simulink library "NAV420Lib"  (Simulink 7.4)
settings: Solver=ode45  StartTime=0.0  StopTime=10.0  RelTol=1e-3
libraries: simulink x25, NAV420Lib x9
settings Model: Creator=djulzz  LastModifiedBy=djulzz

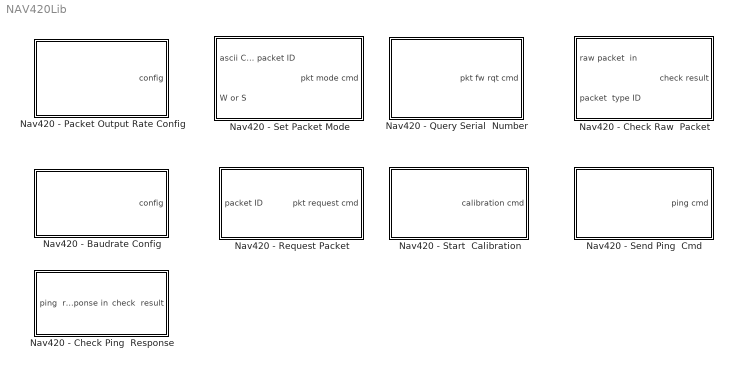
== system NAV420Lib ==
  Nav420 - Baudrate Config : Subsystem  mask{baudrateIndex=9600, SaveConfig=off}
      mask prompts: baudrateIndex "Select the Baudrate (Bauds)"; SaveConfig "Check if the config is to be used at next startup"
      mask StyleString: popup(9600|19200|38400|57600),checkbox
  Nav420 - Check Ping  Response : Subsystem
  Nav420 - Check Raw  Packet : Subsystem
  Nav420 - Packet Output Rate Config : Subsystem  mask{shouldSave=off, output_rate=100}
      mask prompts: shouldSave "Save Ouput Rate for Next Bootup?"; output_rate "Output Rate (Hz)"
      mask StyleString: checkbox,popup(0|2|10|20|25|50|100)
  Nav420 - Query Serial  Number : Subsystem
  Nav420 - Request Packet : Subsystem
  Nav420 - Send Ping  Cmd : Subsystem
  Nav420 - Set Packet Mode : Subsystem
  Nav420 - Start  Calibration : Subsystem

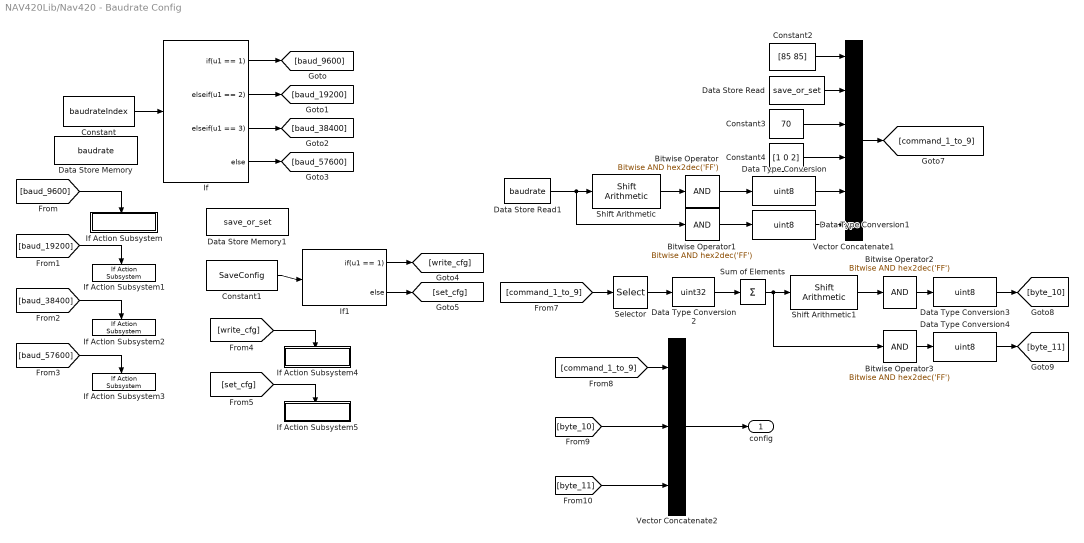
== system NAV420Lib/Nav420 - Baudrate Config ==
  Bitwise Operator{,1..3} (4 alike) : simulink/Logic and Bit Operations/Bitwise Operator  logicop=AND  UseBitMask=on  BitMask=hex2dec('FF')  BitMaskRealWorld=Stored Integer
  Constant : Constant  Value=baudrateIndex  OutDataTypeMode=uint8  OutDataType=fixdt(1, 16)  OutScaling=2^0  OutDataTypeStr=uint8  SampleTime=-1
  Constant1 : Constant  Value=SaveConfig  OutDataTypeMode=uint8  OutDataType=fixdt(1, 16)  OutScaling=2^0  OutDataTypeStr=uint8  SampleTime=-1
  Constant2 : Constant  Value=[85 85]  OutDataTypeMode=uint8  OutDataType=fixdt(1, 16)  OutScaling=2^0  OutDataTypeStr=uint8  SampleTime=-1
  Constant3 : Constant  Value=70  OutDataTypeMode=uint8  OutDataType=fixdt(1, 16)  OutScaling=2^0  OutDataTypeStr=uint8  SampleTime=-1
  Constant4 : Constant  Value=[1 0 2]  OutDataTypeMode=uint8  OutDataType=fixdt(1, 16)  OutScaling=2^0  OutDataTypeStr=uint8  SampleTime=-1
  Data Store Memory : DataStoreMemory  DataStoreName=baudrate  DataType=uint32  OutDataType=fixdt(1, 16)  OutScaling=2^0  OutDataTypeStr=uint32
  Data Store Memory1 : DataStoreMemory  DataStoreName=save_or_set  DataType=uint8  OutDataType=fixdt(1, 16)  OutScaling=2^0  OutDataTypeStr=uint8
  Data Store Read : DataStoreRead  DataStoreName=save_or_set  SampleTime=-1
  Data Store Read1 : DataStoreRead  DataStoreName=baudrate  SampleTime=0
  Data Type Conversion{,1,3..4} (4 alike) : DataTypeConversion  OutDataTypeMode=uint8  OutDataType=fixdt(1, 16)  OutScaling=2^0  OutDataTypeStr=uint8  RndMeth=Nearest
  Data Type Conversion2 : DataTypeConversion  OutDataTypeMode=uint32  OutDataType=fixdt(1, 16)  OutScaling=2^0  OutDataTypeStr=uint32  RndMeth=Nearest
  If : If  IfExpression=u1 == 1  ElseIfExpressions=u1 == 2, u1 == 3
  If Action Subsystem : Subsystem  TreatAsAtomicUnit=on
  If Action Subsystem1 : NAV420Lib/Nav420 - Baudrate Config/If Action Subsystem  SystemSampleTime=-1
      link override Constant: Value=1
      link override Data Store Write: DataStoreName=baudrate
  If Action Subsystem2 : NAV420Lib/Nav420 - Baudrate Config/If Action Subsystem  SystemSampleTime=-1
      link override Constant: Value=2
      link override Data Store Write: DataStoreName=baudrate
  If Action Subsystem3 : NAV420Lib/Nav420 - Baudrate Config/If Action Subsystem  SystemSampleTime=-1
      link override Constant: Value=3
      link override Data Store Write: DataStoreName=baudrate
  If Action Subsystem4 : Subsystem  AncestorBlock=|  TreatAsAtomicUnit=on
      | NAV420Lib/Nav420 - Baudrate
      | Config/If Action
      | Subsystem
  If Action Subsystem5 : Subsystem  AncestorBlock=|  TreatAsAtomicUnit=on
      | NAV420Lib/Nav420 - Baudrate
      | Config/If Action
      | Subsystem
  If1 : If  IfExpression=u1 == 1
  Selector : Selector  InputPortWidth=9  IndexOptions=Index vector (dialog)  Indices=[3 4 5 6 7 8 9]  OutputSizes=1
  Shift Arithmetic : simulink/Logic and Bit Operations/Shift Arithmetic  SystemSampleTime=-1  nBitShiftRight=8  nBinPtShiftRight=0
  Shift Arithmetic1 : simulink/Logic and Bit Operations/Shift Arithmetic  SystemSampleTime=-1  nBitShiftRight=8  nBinPtShiftRight=0
  Sum of Elements : Sum  Inputs=+  OutDataType=fixdt(1, 16)  OutScaling=2^-10
  Vector Concatenate1 : Concatenate  NumInputs=6  Mode=Vector
  Vector Concatenate2 : Concatenate  NumInputs=3  Mode=Vector
  config : Outport  DataType=uint8  OutDataType=fixdt(1, 16)  OutScaling=2^0  OutDataTypeStr=uint8
  wires:
  Constant/1 -> If/1
  If/1 -> [baud_9600]
  If/2 -> [baud_19200]
  If/3 -> [baud_38400]
  If/4 -> [baud_57600]
  [baud_9600] -> If Action Subsystem/Action
  [baud_19200] -> If Action Subsystem1/Action
  [baud_38400] -> If Action Subsystem2/Action
  [baud_57600] -> If Action Subsystem3/Action
  Data Store Read1/1 -> Shift Arithmetic/1, Bitwise Operator1/1
  Shift Arithmetic/1 -> Bitwise Operator/1
  Bitwise Operator1/1 -> Data Type Conversion1/1
  Bitwise Operator/1 -> Data Type Conversion/1
  Constant1/1 -> If1/1
  If1/2 -> [set_cfg]
  If1/1 -> [write_cfg]
  [write_cfg] -> If Action Subsystem4/Action
  [set_cfg] -> If Action Subsystem5/Action
  Constant2/1 -> Vector Concatenate1/1
  Data Store Read/1 -> Vector Concatenate1/2
  Constant3/1 -> Vector Concatenate1/3
  Constant4/1 -> Vector Concatenate1/4
  Data Type Conversion/1 -> Vector Concatenate1/5
  Data Type Conversion1/1 -> Vector Concatenate1/6
  Vector Concatenate1/1 -> [command_1_to_9]
  Selector/1 -> Data Type Conversion2/1
  Data Type Conversion2/1 -> Sum of Elements/1
  Shift Arithmetic1/1 -> Bitwise Operator2/1
  Bitwise Operator2/1 -> Data Type Conversion3/1
  Sum of Elements/1 -> Shift Arithmetic1/1, Bitwise Operator3/1
  [command_1_to_9] -> Selector/1
  Data Type Conversion3/1 -> [byte_10]
  Bitwise Operator3/1 -> Data Type Conversion4/1
  Data Type Conversion4/1 -> [byte_11]
  [command_1_to_9] -> Vector Concatenate2/1
  [byte_10] -> Vector Concatenate2/2
  [byte_11] -> Vector Concatenate2/3
  Vector Concatenate2/1 -> config/1

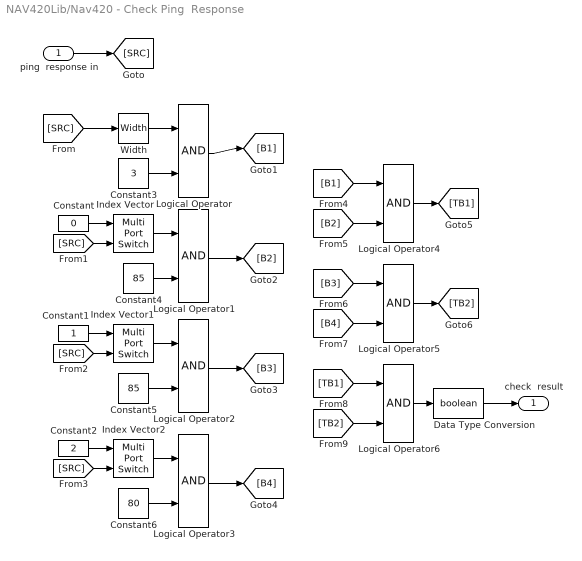
== system NAV420Lib/Nav420 - Check Ping  Response ==
  ping  response in : Inport  DataType=uint8  OutDataType=fixdt(1, 16)  OutScaling=2^0  OutDataTypeStr=uint8
  Constant : Constant  Value=0  OutDataType=fixdt(1, 16)  OutScaling=2^0  SampleTime=-1
  Constant1 : Constant  OutDataType=fixdt(1, 16)  OutScaling=2^0  SampleTime=-1
  Constant2 : Constant  Value=2  OutDataType=fixdt(1, 16)  OutScaling=2^0  SampleTime=-1
  Constant3 : Constant  Value=3  OutDataTypeMode=uint8  OutDataType=fixdt(1, 16)  OutScaling=2^0  OutDataTypeStr=uint8  SampleTime=-1
  Constant4 : Constant  Value=85  OutDataTypeMode=uint8  OutDataType=fixdt(1, 16)  OutScaling=2^0  OutDataTypeStr=uint8  SampleTime=-1
  Constant5 : Constant  Value=85  OutDataTypeMode=uint8  OutDataType=fixdt(1, 16)  OutScaling=2^0  OutDataTypeStr=uint8  SampleTime=-1
  Constant6 : Constant  Value=80  OutDataTypeMode=uint8  OutDataType=fixdt(1, 16)  OutScaling=2^0  OutDataTypeStr=uint8  SampleTime=-1
  Data Type Conversion : DataTypeConversion  OutDataTypeMode=boolean  OutDataType=fixdt(1, 16)  OutScaling=2^0  OutDataTypeStr=boolean
  Index Vector : MultiPortSwitch  Inputs=1  zeroidx=on  OutDataType=fixdt(1, 16)  OutScaling=2^0
  Index Vector1 : MultiPortSwitch  Inputs=1  zeroidx=on  OutDataType=fixdt(1, 16)  OutScaling=2^0
  Index Vector2 : MultiPortSwitch  Inputs=1  zeroidx=on  OutDataType=fixdt(1, 16)  OutScaling=2^0
  Logical Operator{,1..6} (7 alike) : Logic  AllPortsSameDT=off  OutDataTypeMode=boolean  LogicDataType=fixdt(0, 8)  OutDataTypeStr=boolean
  Width : Width
  check  result : Outport  DataType=boolean  OutDataType=fixdt(1, 16)  OutScaling=2^0  OutDataTypeStr=boolean
  wires:
  ping  response in/1 -> [SRC]
  [SRC] -> Width/1
  [SRC] -> Index Vector2/2
  [SRC] -> Index Vector1/2
  [SRC] -> Index Vector/2
  Constant/1 -> Index Vector/1
  Constant1/1 -> Index Vector1/1
  Constant2/1 -> Index Vector2/1
  Width/1 -> Logical Operator/1
  Constant3/1 -> Logical Operator/2
  Index Vector/1 -> Logical Operator1/1
  Constant4/1 -> Logical Operator1/2
  Constant5/1 -> Logical Operator2/2
  Index Vector1/1 -> Logical Operator2/1
  Constant6/1 -> Logical Operator3/2
  Index Vector2/1 -> Logical Operator3/1
  Logical Operator3/1 -> [B4]
  Logical Operator2/1 -> [B3]
  Logical Operator1/1 -> [B2]
  Logical Operator/1 -> [B1]
  [B2] -> Logical Operator4/2
  [B1] -> Logical Operator4/1
  [B4] -> Logical Operator5/2
  [B3] -> Logical Operator5/1
  Logical Operator5/1 -> [TB2]
  Logical Operator4/1 -> [TB1]
  [TB2] -> Logical Operator6/2
  [TB1] -> Logical Operator6/1
  Logical Operator6/1 -> Data Type Conversion/1
  Data Type Conversion/1 -> check  result/1

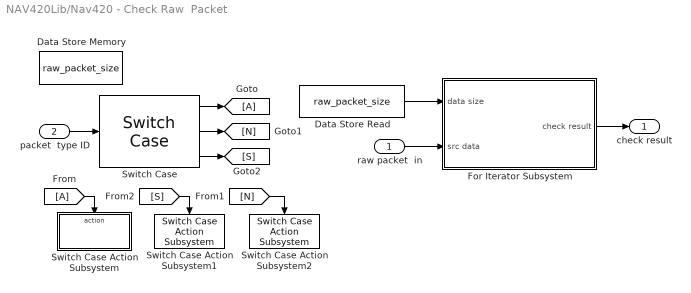
== system NAV420Lib/Nav420 - Check Raw  Packet ==
  raw packet  in : Inport  DataType=uint8  OutDataType=fixdt(1, 16)  OutScaling=2^0  OutDataTypeStr=uint8
  packet  type ID : Inport  Port=2  DataType=int8  OutDataType=fixdt(1, 16)  OutScaling=2^0  OutDataTypeStr=int8
  Data Store Memory : DataStoreMemory  DataStoreName=raw_packet_size  DataType=uint8  OutDataType=fixdt(1, 16)  OutScaling=2^0  OutDataTypeStr=uint8
  Data Store Read : DataStoreRead  DataStoreName=raw_packet_size  SampleTime=-1
  For Iterator Subsystem : Subsystem  TreatAsAtomicUnit=on
  Switch Case : SwitchCase  CaseConditions={65,78}
  Switch Case Action Subsystem : Subsystem  TreatAsAtomicUnit=on
  Switch Case Action Subsystem1 : NAV420Lib/Nav420 - Check Raw  Packet/Switch Case Action Subsystem  SystemSampleTime=-1
  Switch Case Action Subsystem2 : NAV420Lib/Nav420 - Check Raw  Packet/Switch Case Action Subsystem  SystemSampleTime=-1
      link override Constant: Value=37
  check result : Outport  DataType=boolean  OutDataType=fixdt(1, 16)  OutScaling=2^0  OutDataTypeStr=boolean
  wires:
  packet  type ID/1 -> Switch Case/1
  Switch Case/1 -> [A]
  Switch Case/2 -> [N]
  Switch Case/3 -> [S]
  [A] -> Switch Case Action Subsystem/Action
  [S] -> Switch Case Action Subsystem1/Action
  [N] -> Switch Case Action Subsystem2/Action
  Data Store Read/1 -> For Iterator Subsystem/1(data size)
  raw packet  in/1 -> For Iterator Subsystem/2(src data)
  For Iterator Subsystem/1(check result) -> check result/1

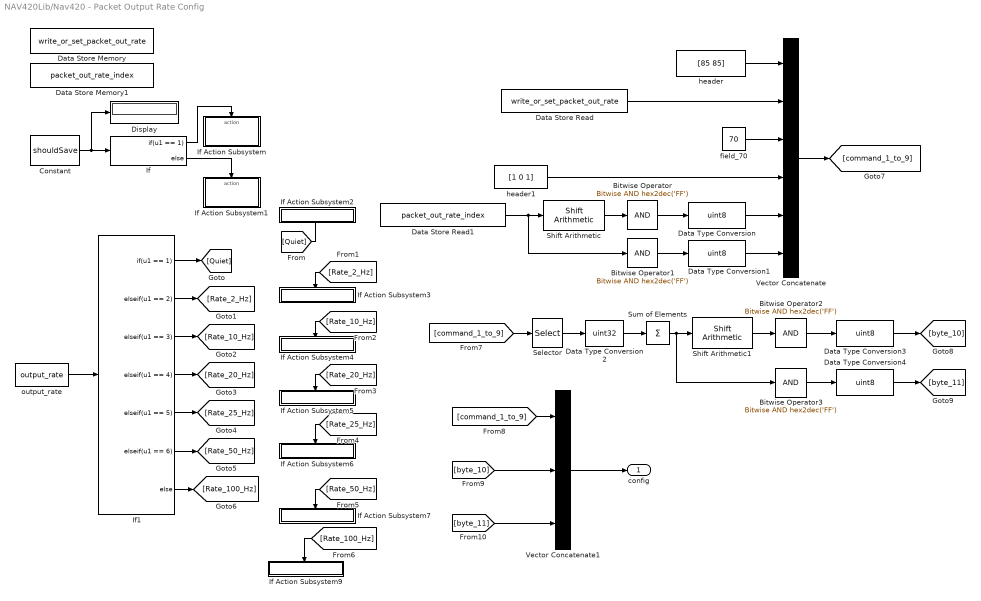
== system NAV420Lib/Nav420 - Packet Output Rate Config ==
  Bitwise Operator{,1..3} (4 alike) : simulink/Logic and Bit Operations/Bitwise Operator  logicop=AND  UseBitMask=on  BitMask=hex2dec('FF')  BitMaskRealWorld=Stored Integer
  Constant : Constant  Value=shouldSave  OutDataTypeMode=int32  OutDataType=fixdt(1, 16)  OutScaling=2^0  OutDataTypeStr=int32  SampleTime=-1
  Data Store Memory : DataStoreMemory  DataStoreName=write_or_set_packet_out_rate  DataType=uint8  OutDataType=fixdt(1, 16)  OutScaling=2^0  OutDataTypeStr=uint8
  Data Store Memory1 : DataStoreMemory  DataStoreName=packet_out_rate_index  DataType=uint8  OutDataType=fixdt(1, 16)  OutScaling=2^0  OutDataTypeStr=uint8
  Data Store Read : DataStoreRead  DataStoreName=write_or_set_packet_out_rate  SampleTime=-1
  Data Store Read1 : DataStoreRead  DataStoreName=packet_out_rate_index  SampleTime=-1
  Data Type Conversion{,1,3..4} (4 alike) : DataTypeConversion  OutDataTypeMode=uint8  OutDataType=fixdt(1, 16)  OutScaling=2^0  OutDataTypeStr=uint8  RndMeth=Nearest
  Data Type Conversion2 : DataTypeConversion  OutDataTypeMode=uint32  OutDataType=fixdt(1, 16)  OutScaling=2^0  OutDataTypeStr=uint32  RndMeth=Nearest
  Display : Display
  If : If  IfExpression=u1 == 1
  If Action Subsystem : Subsystem  TreatAsAtomicUnit=on
  If Action Subsystem1 : Subsystem  TreatAsAtomicUnit=on
  If Action Subsystem2 : Subsystem  TreatAsAtomicUnit=on
  If Action Subsystem3 : Subsystem  TreatAsAtomicUnit=on
  If Action Subsystem4 : Subsystem  TreatAsAtomicUnit=on
  If Action Subsystem5 : Subsystem  TreatAsAtomicUnit=on
  If Action Subsystem6 : Subsystem  TreatAsAtomicUnit=on
  If Action Subsystem7 : Subsystem  TreatAsAtomicUnit=on
  If Action Subsystem9 : Subsystem  TreatAsAtomicUnit=on
  If1 : If  IfExpression=u1 == 1  ElseIfExpressions=u1 == 2, u1 == 3, u1 == 4, u1 == 5, u1 == 6
  Selector : Selector  InputPortWidth=9  IndexOptions=Index vector (dialog)  Indices=[3 4 5 6 7 8 9]  OutputSizes=1
  Shift Arithmetic : simulink/Logic and Bit Operations/Shift Arithmetic  SystemSampleTime=-1  nBitShiftRight=8  nBinPtShiftRight=0
  Shift Arithmetic1 : simulink/Logic and Bit Operations/Shift Arithmetic  SystemSampleTime=-1  nBitShiftRight=8  nBinPtShiftRight=0
  Sum of Elements : Sum  Inputs=+  OutDataType=fixdt(1, 16)  OutScaling=2^-10
  Vector Concatenate : Concatenate  NumInputs=6  Mode=Vector
  Vector Concatenate1 : Concatenate  NumInputs=3  Mode=Vector
  field_70 : Constant  Value=70  OutDataTypeMode=uint8  OutDataType=fixdt(1, 16)  OutScaling=2^0  OutDataTypeStr=uint8  SampleTime=-1
  header : Constant  Value=[85 85]  OutDataTypeMode=uint8  OutDataType=fixdt(1, 16)  OutScaling=2^0  OutDataTypeStr=uint8  SampleTime=-1
  header1 : Constant  Value=[1 0 1]  OutDataTypeMode=uint8  OutDataType=fixdt(1, 16)  OutScaling=2^0  OutDataTypeStr=uint8  SampleTime=-1
  output_rate : Constant  Value=output_rate  OutDataTypeMode=uint8  OutDataType=fixdt(1, 16)  OutScaling=2^0  OutDataTypeStr=uint8  SampleTime=-1
  config : Outport  DataType=uint8  OutDataType=fixdt(1, 16)  OutScaling=2^0  OutDataTypeStr=uint8
  wires:
  Constant/1 -> If/1, Display/1
  If/2 -> If Action Subsystem1/Action
  header/1 -> Vector Concatenate/1
  If/1 -> If Action Subsystem/Action
  Data Store Read/1 -> Vector Concatenate/2
  field_70/1 -> Vector Concatenate/3
  header1/1 -> Vector Concatenate/4
  output_rate/1 -> If1/1
  Data Store Read1/1 -> Shift Arithmetic/1, Bitwise Operator1/1
  Shift Arithmetic/1 -> Bitwise Operator/1
  Bitwise Operator1/1 -> Data Type Conversion1/1
  Bitwise Operator/1 -> Data Type Conversion/1
  Data Type Conversion/1 -> Vector Concatenate/5
  Data Type Conversion1/1 -> Vector Concatenate/6
  If1/1 -> [Quiet]
  [Quiet] -> If Action Subsystem2/Action
  If1/2 -> [Rate_2_Hz]
  [Rate_2_Hz] -> If Action Subsystem3/Action
  If1/3 -> [Rate_10_Hz]
  [Rate_10_Hz] -> If Action Subsystem4/Action
  If1/4 -> [Rate_20_Hz]
  [Rate_20_Hz] -> If Action Subsystem5/Action
  If1/5 -> [Rate_25_Hz]
  [Rate_25_Hz] -> If Action Subsystem6/Action
  If1/6 -> [Rate_50_Hz]
  [Rate_50_Hz] -> If Action Subsystem7/Action
  If1/7 -> [Rate_100_Hz]
  [Rate_100_Hz] -> If Action Subsystem9/Action
  Selector/1 -> Data Type Conversion2/1
  Data Type Conversion2/1 -> Sum of Elements/1
  Shift Arithmetic1/1 -> Bitwise Operator2/1
  Bitwise Operator2/1 -> Data Type Conversion3/1
  Sum of Elements/1 -> Shift Arithmetic1/1, Bitwise Operator3/1
  Bitwise Operator3/1 -> Data Type Conversion4/1
  Vector Concatenate/1 -> [command_1_to_9]
  [command_1_to_9] -> Selector/1
  Data Type Conversion3/1 -> [byte_10]
  Data Type Conversion4/1 -> [byte_11]
  [command_1_to_9] -> Vector Concatenate1/1
  [byte_10] -> Vector Concatenate1/2
  [byte_11] -> Vector Concatenate1/3
  Vector Concatenate1/1 -> config/1

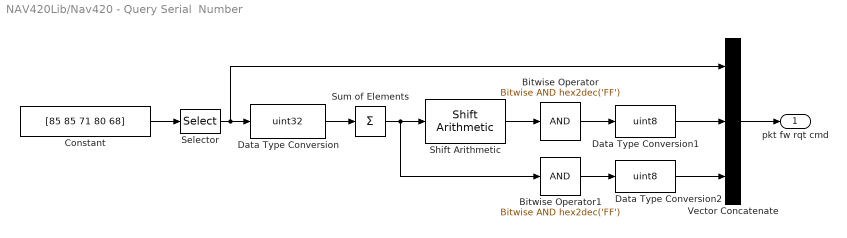
== system NAV420Lib/Nav420 - Query Serial  Number ==
  Bitwise Operator : simulink/Logic and Bit Operations/Bitwise Operator  logicop=AND  UseBitMask=on  BitMask=hex2dec('FF')  BitMaskRealWorld=Stored Integer
  Bitwise Operator1 : simulink/Logic and Bit Operations/Bitwise Operator  logicop=AND  UseBitMask=on  BitMask=hex2dec('FF')  BitMaskRealWorld=Stored Integer
  Constant : Constant  Value=[85 85 71 80 68]  OutDataTypeMode=uint8  OutDataType=fixdt(1, 16)  OutScaling=2^0  OutDataTypeStr=uint8
  Data Type Conversion : DataTypeConversion  OutDataTypeMode=uint32  OutDataType=fixdt(1, 16)  OutScaling=2^0  OutDataTypeStr=uint32
  Data Type Conversion1 : DataTypeConversion  OutDataTypeMode=uint8  OutDataType=fixdt(1, 16)  OutScaling=2^0  OutDataTypeStr=uint8
  Data Type Conversion2 : DataTypeConversion  OutDataTypeMode=uint8  OutDataType=fixdt(1, 16)  OutScaling=2^0  OutDataTypeStr=uint8
  Selector : Selector  InputPortWidth=5  IndexOptions=Index vector (dialog)  Indices=[3 4 5]  OutputSizes=1
  Shift Arithmetic : simulink/Logic and Bit Operations/Shift Arithmetic  SystemSampleTime=-1  nBitShiftRight=8  nBinPtShiftRight=0
  Sum of Elements : Sum  Inputs=+  OutDataType=fixdt(1, 16)  OutScaling=2^-10
  Vector Concatenate : Concatenate  NumInputs=3  Mode=Vector
  pkt fw rqt cmd : Outport  OutDataType=fixdt(1, 16)  OutScaling=2^0
  wires:
  Constant/1 -> Selector/1
  Selector/1 -> Data Type Conversion/1, Vector Concatenate/1
  Data Type Conversion/1 -> Sum of Elements/1
  Sum of Elements/1 -> Shift Arithmetic/1, Bitwise Operator1/1
  Shift Arithmetic/1 -> Bitwise Operator/1
  Bitwise Operator/1 -> Data Type Conversion1/1
  Bitwise Operator1/1 -> Data Type Conversion2/1
  Data Type Conversion2/1 -> Vector Concatenate/3
  Data Type Conversion1/1 -> Vector Concatenate/2
  Vector Concatenate/1 -> pkt fw rqt cmd/1

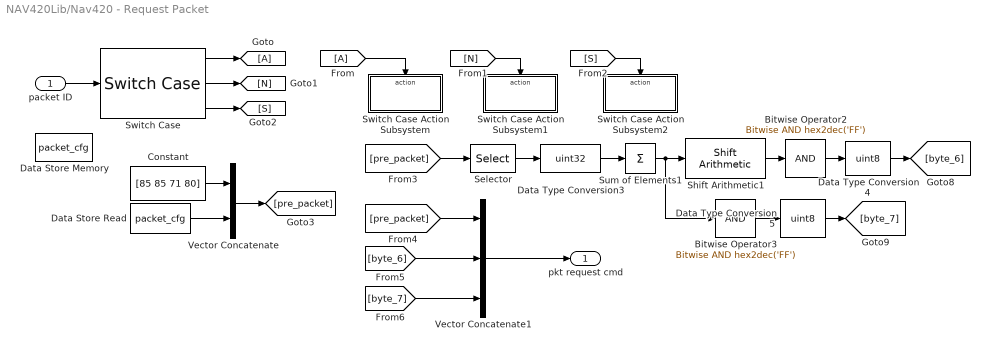
== system NAV420Lib/Nav420 - Request Packet ==
  packet ID : Inport  DataType=int8  OutDataType=fixdt(1, 16)  OutScaling=2^0  OutDataTypeStr=int8
  Bitwise Operator2 : simulink/Logic and Bit Operations/Bitwise Operator  logicop=AND  UseBitMask=on  BitMask=hex2dec('FF')  BitMaskRealWorld=Stored Integer
  Bitwise Operator3 : simulink/Logic and Bit Operations/Bitwise Operator  logicop=AND  UseBitMask=on  BitMask=hex2dec('FF')  BitMaskRealWorld=Stored Integer
  Constant : Constant  Value=[85 85 71 80]  OutDataTypeMode=uint8  OutDataType=fixdt(1, 16)  OutScaling=2^0  OutDataTypeStr=uint8  SampleTime=-1
  Data Store Memory : DataStoreMemory  DataStoreName=packet_cfg  DataType=uint8  OutDataType=fixdt(1, 16)  OutScaling=2^0  OutDataTypeStr=uint8
  Data Store Read : DataStoreRead  DataStoreName=packet_cfg  SampleTime=-1
  Data Type Conversion3 : DataTypeConversion  OutDataTypeMode=uint32  OutDataType=fixdt(1, 16)  OutScaling=2^0  OutDataTypeStr=uint32  RndMeth=Nearest
  Data Type Conversion4 : DataTypeConversion  OutDataTypeMode=uint8  OutDataType=fixdt(1, 16)  OutScaling=2^0  OutDataTypeStr=uint8  RndMeth=Nearest
  Data Type Conversion5 : DataTypeConversion  OutDataTypeMode=uint8  OutDataType=fixdt(1, 16)  OutScaling=2^0  OutDataTypeStr=uint8  RndMeth=Nearest
  Selector : Selector  InputPortWidth=5  IndexOptions=Index vector (dialog)  Indices=[3 4 5]  OutputSizes=1
  Shift Arithmetic1 : simulink/Logic and Bit Operations/Shift Arithmetic  SystemSampleTime=-1  nBitShiftRight=8  nBinPtShiftRight=0
  Sum of Elements1 : Sum  Inputs=+  OutDataType=fixdt(1, 16)  OutScaling=2^-10
  Switch Case : SwitchCase  CaseConditions={65,78}
  Switch Case Action Subsystem : Subsystem  TreatAsAtomicUnit=on
  Switch Case Action Subsystem1 : Subsystem  TreatAsAtomicUnit=on
  Switch Case Action Subsystem2 : Subsystem  TreatAsAtomicUnit=on
  Vector Concatenate : Concatenate  Mode=Vector
  Vector Concatenate1 : Concatenate  NumInputs=3  Mode=Vector
  pkt request cmd : Outport  DataType=uint8  OutDataType=fixdt(1, 16)  OutScaling=2^0  OutDataTypeStr=uint8
  wires:
  packet ID/1 -> Switch Case/1
  Switch Case/1 -> [A]
  Switch Case/2 -> [N]
  Switch Case/3 -> [S]
  [A] -> Switch Case Action Subsystem/Action
  [N] -> Switch Case Action Subsystem1/Action
  [S] -> Switch Case Action Subsystem2/Action
  Constant/1 -> Vector Concatenate/1
  Data Store Read/1 -> Vector Concatenate/2
  Vector Concatenate/1 -> [pre_packet]
  [pre_packet] -> Selector/1
  Selector/1 -> Data Type Conversion3/1
  Shift Arithmetic1/1 -> Bitwise Operator2/1
  Bitwise Operator2/1 -> Data Type Conversion4/1
  Bitwise Operator3/1 -> Data Type Conversion5/1
  Data Type Conversion4/1 -> [byte_6]
  Data Type Conversion5/1 -> [byte_7]
  Sum of Elements1/1 -> Shift Arithmetic1/1, Bitwise Operator3/1
  Data Type Conversion3/1 -> Sum of Elements1/1
  [pre_packet] -> Vector Concatenate1/1
  [byte_6] -> Vector Concatenate1/2
  [byte_7] -> Vector Concatenate1/3
  Vector Concatenate1/1 -> pkt request cmd/1

== system NAV420Lib/Nav420 - Send Ping  Cmd ==
  Constant : Constant  Value=[85 85 80 75]  OutDataTypeMode=uint8  OutDataType=fixdt(1, 16)  OutScaling=2^0  OutDataTypeStr=uint8  SampleTime=-1
  ping cmd : Outport  DataType=uint8  OutDataType=fixdt(1, 16)  OutScaling=2^0  OutDataTypeStr=uint8
  wires:
  Constant/1 -> ping cmd/1

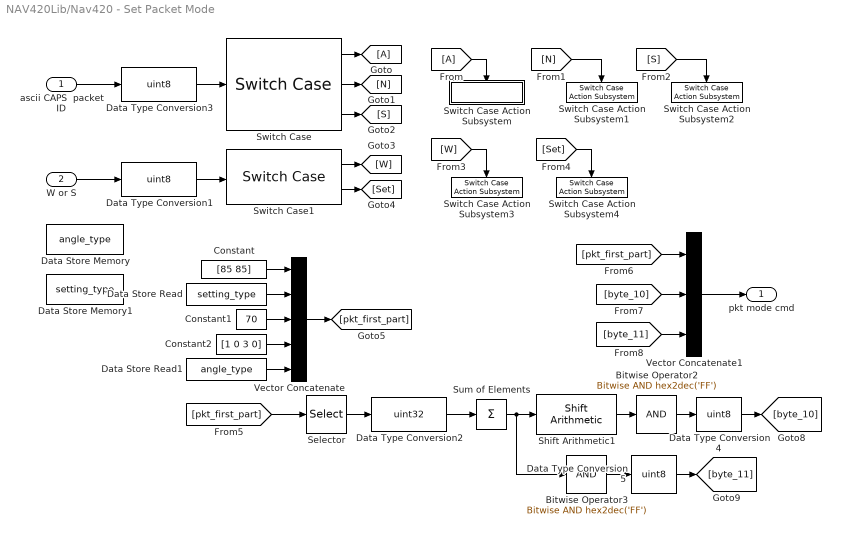
== system NAV420Lib/Nav420 - Set Packet Mode ==
  ascii CAPS  packet ID : Inport  DataType=int8  OutDataType=fixdt(1, 16)  OutScaling=2^0  OutDataTypeStr=int8
  W or S : Inport  Port=2  DataType=int8  OutDataType=fixdt(1, 16)  OutScaling=2^0  OutDataTypeStr=int8
  Bitwise Operator2 : simulink/Logic and Bit Operations/Bitwise Operator  logicop=AND  UseBitMask=on  BitMask=hex2dec('FF')  BitMaskRealWorld=Stored Integer
  Bitwise Operator3 : simulink/Logic and Bit Operations/Bitwise Operator  logicop=AND  UseBitMask=on  BitMask=hex2dec('FF')  BitMaskRealWorld=Stored Integer
  Constant : Constant  Value=[85 85]  OutDataTypeMode=uint8  OutDataType=fixdt(1, 16)  OutScaling=2^0  OutDataTypeStr=uint8  SampleTime=-1
  Constant1 : Constant  Value=70  OutDataTypeMode=uint8  OutDataType=fixdt(1, 16)  OutScaling=2^0  OutDataTypeStr=uint8  SampleTime=-1
  Constant2 : Constant  Value=[1 0 3 0]  OutDataTypeMode=uint8  OutDataType=fixdt(1, 16)  OutScaling=2^0  OutDataTypeStr=uint8  SampleTime=-1
  Data Store Memory : DataStoreMemory  DataStoreName=angle_type  DataType=uint8  OutDataType=fixdt(1, 16)  OutScaling=2^0  OutDataTypeStr=uint8
  Data Store Memory1 : DataStoreMemory  DataStoreName=setting_type  DataType=uint8  OutDataType=fixdt(1, 16)  OutScaling=2^0  OutDataTypeStr=uint8
  Data Store Read : DataStoreRead  DataStoreName=setting_type  SampleTime=-1
  Data Store Read1 : DataStoreRead  DataStoreName=angle_type  SampleTime=-1
  Data Type Conversion{1,3..5} (4 alike) : DataTypeConversion  OutDataTypeMode=uint8  OutDataType=fixdt(1, 16)  OutScaling=2^0  OutDataTypeStr=uint8  RndMeth=Nearest
  Data Type Conversion2 : DataTypeConversion  OutDataTypeMode=uint32  OutDataType=fixdt(1, 16)  OutScaling=2^0  OutDataTypeStr=uint32  RndMeth=Nearest
  Selector : Selector  InputPortWidth=9  IndexOptions=Index vector (dialog)  Indices=[3 4 5 6 7 8 9]  OutputSizes=1
  Shift Arithmetic1 : simulink/Logic and Bit Operations/Shift Arithmetic  SystemSampleTime=-1  nBitShiftRight=8  nBinPtShiftRight=0
  Sum of Elements : Sum  Inputs=+  OutDataType=fixdt(1, 16)  OutScaling=2^-10
  Switch Case : SwitchCase  CaseConditions={65,78}
  Switch Case Action Subsystem : Subsystem  TreatAsAtomicUnit=on
  Switch Case Action Subsystem1 : NAV420Lib/Nav420 - Set Packet Mode/Switch Case Action Subsystem  SystemSampleTime=-1
      link override Constant1: Value=78
  Switch Case Action Subsystem2 : NAV420Lib/Nav420 - Set Packet Mode/Switch Case Action Subsystem  SystemSampleTime=-1
      link override Constant1: Value=83
  Switch Case Action Subsystem3 : NAV420Lib/Nav420 - Set Packet Mode/Switch Case Action Subsystem  SystemSampleTime=-1
      link override Constant1: Value=87
      link override Data Store Write: DataStoreName=setting_type
  Switch Case Action Subsystem4 : NAV420Lib/Nav420 - Set Packet Mode/Switch Case Action Subsystem  SystemSampleTime=-1
      link override Constant1: Value=83
      link override Data Store Write: DataStoreName=setting_type
  Switch Case1 : SwitchCase  CaseConditions={87}
  Vector Concatenate : Concatenate  NumInputs=5  Mode=Vector
  Vector Concatenate1 : Concatenate  NumInputs=3  Mode=Vector
  pkt mode cmd : Outport  DataType=uint8  OutDataType=fixdt(1, 16)  OutScaling=2^0  OutDataTypeStr=uint8
  wires:
  ascii CAPS  packet ID/1 -> Data Type Conversion3/1
  Data Type Conversion3/1 -> Switch Case/1
  Switch Case/3 -> [S]
  Switch Case/2 -> [N]
  Switch Case/1 -> [A]
  W or S/1 -> Data Type Conversion1/1
  Data Type Conversion1/1 -> Switch Case1/1
  Switch Case1/1 -> [W]
  Switch Case1/2 -> [Set]
  [A] -> Switch Case Action Subsystem/Action
  [N] -> Switch Case Action Subsystem1/Action
  [S] -> Switch Case Action Subsystem2/Action
  [W] -> Switch Case Action Subsystem3/Action
  [Set] -> Switch Case Action Subsystem4/Action
  Constant/1 -> Vector Concatenate/1
  Data Store Read/1 -> Vector Concatenate/2
  Constant1/1 -> Vector Concatenate/3
  Constant2/1 -> Vector Concatenate/4
  Data Store Read1/1 -> Vector Concatenate/5
  Vector Concatenate/1 -> [pkt_first_part]
  [pkt_first_part] -> Selector/1
  Selector/1 -> Data Type Conversion2/1
  Data Type Conversion2/1 -> Sum of Elements/1
  Shift Arithmetic1/1 -> Bitwise Operator2/1
  Bitwise Operator2/1 -> Data Type Conversion4/1
  Bitwise Operator3/1 -> Data Type Conversion5/1
  Data Type Conversion4/1 -> [byte_10]
  Data Type Conversion5/1 -> [byte_11]
  Sum of Elements/1 -> Shift Arithmetic1/1, Bitwise Operator3/1
  [pkt_first_part] -> Vector Concatenate1/1
  [byte_10] -> Vector Concatenate1/2
  [byte_11] -> Vector Concatenate1/3
  Vector Concatenate1/1 -> pkt mode cmd/1

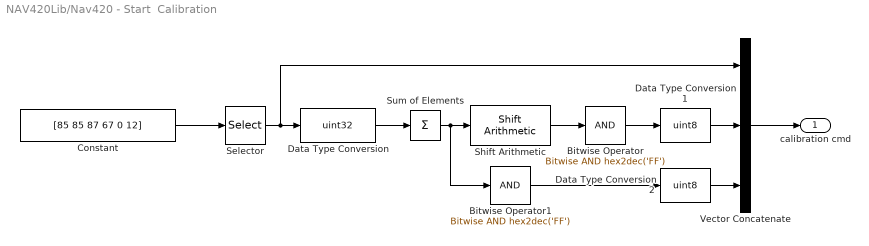
== system NAV420Lib/Nav420 - Start  Calibration ==
  Bitwise Operator : simulink/Logic and Bit Operations/Bitwise Operator  logicop=AND  UseBitMask=on  BitMask=hex2dec('FF')  BitMaskRealWorld=Stored Integer
  Bitwise Operator1 : simulink/Logic and Bit Operations/Bitwise Operator  logicop=AND  UseBitMask=on  BitMask=hex2dec('FF')  BitMaskRealWorld=Stored Integer
  Constant : Constant  Value=[85 85 87 67 0 12]  OutDataTypeMode=uint8  OutDataType=fixdt(1, 16)  OutScaling=2^0  OutDataTypeStr=uint8  SampleTime=-1
  Data Type Conversion : DataTypeConversion  OutDataTypeMode=uint32  OutDataType=fixdt(1, 16)  OutScaling=2^0  OutDataTypeStr=uint32
  Data Type Conversion1 : DataTypeConversion  OutDataTypeMode=uint8  OutDataType=fixdt(1, 16)  OutScaling=2^0  OutDataTypeStr=uint8
  Data Type Conversion2 : DataTypeConversion  OutDataTypeMode=uint8  OutDataType=fixdt(1, 16)  OutScaling=2^0  OutDataTypeStr=uint8
  Selector : Selector  InputPortWidth=6  IndexOptions=Index vector (dialog)  Indices=[3 4 5 6]  OutputSizes=1
  Shift Arithmetic : simulink/Logic and Bit Operations/Shift Arithmetic  SystemSampleTime=-1  nBitShiftRight=8  nBinPtShiftRight=0
  Sum of Elements : Sum  Inputs=+  OutDataType=fixdt(1, 16)  OutScaling=2^-10
  Vector Concatenate : Concatenate  NumInputs=3  Mode=Vector
  calibration cmd : Outport  DataType=uint8  OutDataType=fixdt(1, 16)  OutScaling=2^0  OutDataTypeStr=uint8
  wires:
  Constant/1 -> Selector/1
  Selector/1 -> Data Type Conversion/1, Vector Concatenate/1
  Data Type Conversion/1 -> Sum of Elements/1
  Sum of Elements/1 -> Shift Arithmetic/1, Bitwise Operator1/1
  Shift Arithmetic/1 -> Bitwise Operator/1
  Bitwise Operator/1 -> Data Type Conversion1/1
  Bitwise Operator1/1 -> Data Type Conversion2/1
  Data Type Conversion2/1 -> Vector Concatenate/3
  Data Type Conversion1/1 -> Vector Concatenate/2
  Vector Concatenate/1 -> calibration cmd/1

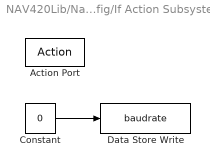
== system NAV420Lib/Nav420 - Baudrate Config/If Action Subsystem ==
  Action Port : ActionPort  PropagateVarSize=During execution  ActionType=then
  Constant : Constant  Value=0  OutDataTypeMode=uint32  OutDataType=fixdt(1, 16)  OutScaling=2^0  OutDataTypeStr=uint32  SampleTime=-1
  Data Store Write : DataStoreWrite  DataStoreName=baudrate  SampleTime=-1
  wires:
  Constant/1 -> Data Store Write/1

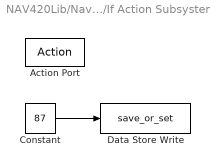
== system NAV420Lib/Nav420 - Baudrate Config/If Action Subsystem4 ==
  Action Port : ActionPort  PropagateVarSize=During execution
  Constant : Constant  Value=87  OutDataTypeMode=uint8  OutDataType=fixdt(1, 16)  OutScaling=2^0  OutDataTypeStr=uint8  SampleTime=-1
  Data Store Write : DataStoreWrite  DataStoreName=save_or_set  SampleTime=-1
  wires:
  Constant/1 -> Data Store Write/1

== system NAV420Lib/Nav420 - Baudrate Config/If Action Subsystem5 ==
  Action Port : ActionPort  PropagateVarSize=During execution
  Constant : Constant  Value=83  OutDataTypeMode=uint8  OutDataType=fixdt(1, 16)  OutScaling=2^0  OutDataTypeStr=uint8  SampleTime=-1
  Data Store Write : DataStoreWrite  DataStoreName=save_or_set  SampleTime=-1
  wires:
  Constant/1 -> Data Store Write/1

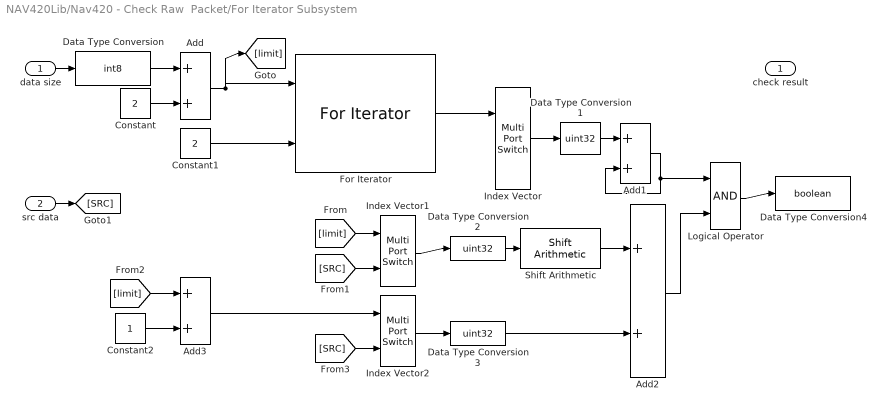
== system NAV420Lib/Nav420 - Check Raw  Packet/For Iterator Subsystem ==
  data size : Inport  DataType=uint8  OutDataType=fixdt(1, 16)  OutScaling=2^0  OutDataTypeStr=uint8
  src data : Inport  Port=2  DataType=uint8  OutDataType=fixdt(1, 16)  OutScaling=2^0  OutDataTypeStr=uint8
  Add{,1..3} (4 alike) : Sum  OutDataType=fixdt(1, 16)  OutScaling=2^-10
  Constant : Constant  Value=2  OutDataTypeMode=int8  OutDataType=fixdt(1, 16)  OutScaling=2^0  OutDataTypeStr=int8  SampleTime=-1
  Constant1 : Constant  Value=2  OutDataTypeMode=int8  OutDataType=fixdt(1, 16)  OutScaling=2^0  OutDataTypeStr=int8  SampleTime=-1
  Constant2 : Constant  OutDataTypeMode=int8  OutDataType=fixdt(1, 16)  OutScaling=2^0  OutDataTypeStr=int8  SampleTime=-1
  Data Type Conversion : DataTypeConversion  OutDataTypeMode=int8  OutDataType=fixdt(1, 16)  OutScaling=2^0  OutDataTypeStr=int8
  Data Type Conversion1 : DataTypeConversion  OutDataTypeMode=uint32  OutDataType=fixdt(1, 16)  OutScaling=2^0  OutDataTypeStr=uint32
  Data Type Conversion2 : DataTypeConversion  OutDataTypeMode=uint32  OutDataType=fixdt(1, 16)  OutScaling=2^0  OutDataTypeStr=uint32
  Data Type Conversion3 : DataTypeConversion  OutDataTypeMode=uint32  OutDataType=fixdt(1, 16)  OutScaling=2^0  OutDataTypeStr=uint32
  Data Type Conversion4 : DataTypeConversion  OutDataTypeMode=boolean  OutDataType=fixdt(1, 16)  OutScaling=2^0  OutDataTypeStr=boolean
  For Iterator : ForIterator  IterationSource=external  ExternalIncrement=on  IndexMode=Zero-based  IterationVariableDataType=int8
  Index Vector : MultiPortSwitch  Inputs=1  zeroidx=on  OutDataTypeMode=uint8  OutDataType=fixdt(1, 16)  OutScaling=2^0  OutDataTypeStr=uint8  InputSameDT=on
  Index Vector1 : MultiPortSwitch  Inputs=1  zeroidx=on  OutDataTypeMode=uint8  OutDataType=fixdt(1, 16)  OutScaling=2^0  OutDataTypeStr=uint8  InputSameDT=on
  Index Vector2 : MultiPortSwitch  Inputs=1  zeroidx=on  OutDataTypeMode=uint8  OutDataType=fixdt(1, 16)  OutScaling=2^0  OutDataTypeStr=uint8  InputSameDT=on
  Logical Operator : Logic  AllPortsSameDT=off  OutDataTypeMode=boolean  LogicDataType=fixdt(0, 8)  OutDataTypeStr=boolean
  Shift Arithmetic : simulink/Logic and Bit Operations/Shift Arithmetic  SystemSampleTime=-1  nBitShiftRight=-8  nBinPtShiftRight=0
  check result : Outport  DataType=boolean  OutDataType=fixdt(1, 16)  OutScaling=2^0  OutDataTypeStr=boolean
  wires:
  data size/1 -> Data Type Conversion/1
  Data Type Conversion/1 -> Add/1
  Constant/1 -> Add/2
  Add/1 -> For Iterator/1, [limit]
  Constant1/1 -> For Iterator/2
  For Iterator/1 -> Index Vector/1
  Index Vector/1 -> Data Type Conversion1/1
  Data Type Conversion1/1 -> Add1/1
  Add1/1 -> Add1/2, Logical Operator/1
  [limit] -> Index Vector1/1
  src data/1 -> [SRC]
  [SRC] -> Index Vector1/2
  [limit] -> Add3/1
  Constant2/1 -> Add3/2
  Add3/1 -> Index Vector2/1
  [SRC] -> Index Vector2/2
  Index Vector1/1 -> Data Type Conversion2/1
  Index Vector2/1 -> Data Type Conversion3/1
  Data Type Conversion2/1 -> Shift Arithmetic/1
  Shift Arithmetic/1 -> Add2/1
  Data Type Conversion3/1 -> Add2/2
  Add2/1 -> Logical Operator/2
  Logical Operator/1 -> Data Type Conversion4/1

== system NAV420Lib/Nav420 - Check Raw  Packet/Switch Case Action Subsystem ==
  Action Port : ActionPort  PropagateVarSize=During execution  ActionType=case
  Constant : Constant  Value=35  OutDataTypeMode=uint8  OutDataType=fixdt(1, 16)  OutScaling=2^0  OutDataTypeStr=uint8  SampleTime=-1
  Data Store Write : DataStoreWrite  DataStoreName=raw_packet_size  SampleTime=-1
  wires:
  Constant/1 -> Data Store Write/1

== system NAV420Lib/Nav420 - Packet Output Rate Config/If Action Subsystem ==
  Action Port : ActionPort  PropagateVarSize=During execution
  Data Store Write : DataStoreWrite  DataStoreName=write_or_set_packet_out_rate  SampleTime=-1
  write : Constant  Value=87  OutDataTypeMode=uint8  OutDataType=fixdt(1, 16)  OutScaling=2^0  OutDataTypeStr=uint8  SampleTime=-1
  wires:
  write/1 -> Data Store Write/1

== system NAV420Lib/Nav420 - Packet Output Rate Config/If Action Subsystem1 ==
  Action Port : ActionPort  PropagateVarSize=During execution
  Data Store Write1 : DataStoreWrite  DataStoreName=write_or_set_packet_out_rate  SampleTime=-1
  set : Constant  Value=83  OutDataTypeMode=uint8  OutDataType=fixdt(1, 16)  OutScaling=2^0  OutDataTypeStr=uint8  SampleTime=-1
  wires:
  set/1 -> Data Store Write1/1

== system NAV420Lib/Nav420 - Packet Output Rate Config/If Action Subsystem2 ==
  Action Port : ActionPort  PropagateVarSize=During execution
  0 = 0 Hz : Constant  Value=0  OutDataTypeMode=uint8  OutDataType=fixdt(1, 16)  OutScaling=2^0  OutDataTypeStr=uint8  SampleTime=-1
  Data Store Write2 : DataStoreWrite  DataStoreName=packet_out_rate_index  SampleTime=-1
  wires:
  0 = 0 Hz/1 -> Data Store Write2/1

== system NAV420Lib/Nav420 - Packet Output Rate Config/If Action Subsystem3 ==
  Action Port : ActionPort  PropagateVarSize=During execution
  50 = 2 Hz : Constant  Value=50  OutDataTypeMode=uint8  OutDataType=fixdt(1, 16)  OutScaling=2^0  OutDataTypeStr=uint8  SampleTime=-1
  Data Store Write2 : DataStoreWrite  DataStoreName=packet_out_rate_index  SampleTime=-1
  wires:
  50 = 2 Hz/1 -> Data Store Write2/1

== system NAV420Lib/Nav420 - Packet Output Rate Config/If Action Subsystem4 ==
  Action Port : ActionPort  PropagateVarSize=During execution
  10 = 10 Hz : Constant  Value=10  OutDataTypeMode=uint8  OutDataType=fixdt(1, 16)  OutScaling=2^0  OutDataTypeStr=uint8  SampleTime=-1
  Data Store Write2 : DataStoreWrite  DataStoreName=packet_out_rate_index  SampleTime=-1
  wires:
  10 = 10 Hz/1 -> Data Store Write2/1

== system NAV420Lib/Nav420 - Packet Output Rate Config/If Action Subsystem5 ==
  Action Port : ActionPort  PropagateVarSize=During execution
  5 = 20 Hz : Constant  Value=5  OutDataTypeMode=uint8  OutDataType=fixdt(1, 16)  OutScaling=2^0  OutDataTypeStr=uint8  SampleTime=-1
  Data Store Write2 : DataStoreWrite  DataStoreName=packet_out_rate_index  SampleTime=-1
  wires:
  5 = 20 Hz/1 -> Data Store Write2/1

== system NAV420Lib/Nav420 - Packet Output Rate Config/If Action Subsystem6 ==
  Action Port : ActionPort  PropagateVarSize=During execution
  4 = 25 Hz : Constant  Value=4  OutDataTypeMode=uint8  OutDataType=fixdt(1, 16)  OutScaling=2^0  OutDataTypeStr=uint8  SampleTime=-1
  Data Store Write2 : DataStoreWrite  DataStoreName=packet_out_rate_index  SampleTime=-1
  wires:
  4 = 25 Hz/1 -> Data Store Write2/1

== system NAV420Lib/Nav420 - Packet Output Rate Config/If Action Subsystem7 ==
  Action Port : ActionPort  PropagateVarSize=During execution
  2 = 50 Hz : Constant  Value=2  OutDataTypeMode=uint8  OutDataType=fixdt(1, 16)  OutScaling=2^0  OutDataTypeStr=uint8  SampleTime=-1
  Data Store Write2 : DataStoreWrite  DataStoreName=packet_out_rate_index  SampleTime=-1
  wires:
  2 = 50 Hz/1 -> Data Store Write2/1

== system NAV420Lib/Nav420 - Packet Output Rate Config/If Action Subsystem9 ==
  Action Port : ActionPort  PropagateVarSize=During execution
  1 = 100 Hz : Constant  OutDataTypeMode=uint8  OutDataType=fixdt(1, 16)  OutScaling=2^0  OutDataTypeStr=uint8  SampleTime=-1
  Data Store Write2 : DataStoreWrite  DataStoreName=packet_out_rate_index  SampleTime=-1
  wires:
  1 = 100 Hz/1 -> Data Store Write2/1

== system NAV420Lib/Nav420 - Request Packet/Switch Case Action Subsystem ==
  Action Port : ActionPort  PropagateVarSize=During execution  ActionType=case
  Constant : Constant  Value=65  OutDataTypeMode=uint8  OutDataType=fixdt(1, 16)  OutScaling=2^0  OutDataTypeStr=uint8  SampleTime=-1
  Data Store Write : DataStoreWrite  DataStoreName=packet_cfg  SampleTime=-1
  wires:
  Constant/1 -> Data Store Write/1

== system NAV420Lib/Nav420 - Request Packet/Switch Case Action Subsystem1 ==
  Action Port : ActionPort  PropagateVarSize=During execution  ActionType=case
  Constant : Constant  Value=78  OutDataTypeMode=uint8  OutDataType=fixdt(1, 16)  OutScaling=2^0  OutDataTypeStr=uint8  SampleTime=-1
  Data Store Write : DataStoreWrite  DataStoreName=packet_cfg  SampleTime=-1
  wires:
  Constant/1 -> Data Store Write/1

== system NAV420Lib/Nav420 - Request Packet/Switch Case Action Subsystem2 ==
  Action Port : ActionPort  PropagateVarSize=During execution  ActionType=default
  Constant : Constant  Value=83  OutDataTypeMode=uint8  OutDataType=fixdt(1, 16)  OutScaling=2^0  OutDataTypeStr=uint8  SampleTime=-1
  Data Store Write : DataStoreWrite  DataStoreName=packet_cfg  SampleTime=-1
  wires:
  Constant/1 -> Data Store Write/1

== system NAV420Lib/Nav420 - Set Packet Mode/Switch Case Action Subsystem ==
  Action Port : ActionPort  PropagateVarSize=During execution  ActionType=case
  Constant1 : Constant  Value=65  OutDataTypeMode=uint8  OutDataType=fixdt(1, 16)  OutScaling=2^0  OutDataTypeStr=uint8  SampleTime=-1
  Data Store Write : DataStoreWrite  DataStoreName=angle_type  SampleTime=-1
  wires:
  Constant1/1 -> Data Store Write/1
